simulink model "canal_aquatico_v2"  (R2014a)
settings: Solver=ode45  StartTime=0.0  StopTime=10.0  RelTol=1e-3
libraries: dspsigops x6
settings Model: Creator=andre  LastModifiedBy=andre

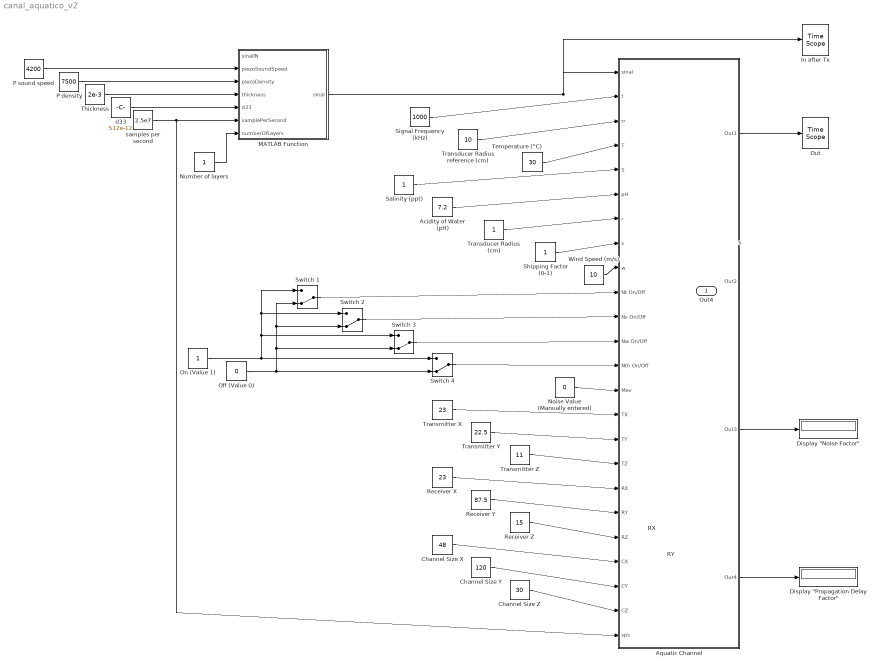
== system canal_aquatico_v2 ==
  s : Inport
  RX : Inport  Port=2
  RY : Inport  Port=3
  Acidity of Water (pH) : Constant  Value=7.2
  Aquatic Channel : Subsystem
  Channel Size X : Constant  Value=48
  Channel Size Y : Constant  Value=120
  Channel Size Z : Constant  Value=30
  "Display \"Propagation Delay Factor\"" : Display
  "Display \"Noise Factor\"" : Display
  In after Tx : TimeScope  DefaultConfigurationName=spbscopes.TimeScopeBlockCfg
  MATLAB Function : MATLAB Function  TreatAsAtomicUnit=on
  Noise Value (Manually entered) : Constant  Value=0
  Number of layers : Constant
  Off (Value 0) : Constant  Value=0
  On (Value 1) : Constant
  Out : TimeScope  DefaultConfigurationName=spbscopes.TimeScopeBlockCfg
  P density : Constant  Value=7500
  P sound speed : Constant  Value=4200
  Receiver X : Constant  Value=23
  Receiver Y : Constant  Value=87.5
  Receiver Z : Constant  Value=15
  Salinity (ppt) : Constant
  Shipping Factor (0-1) : Constant
  Signal Frequency (kHz) : Constant  Value=1000
  Switch {1..4} (4 alike) : ManualSwitch  CurrentSetting=0
  Temperature (°C) : Constant  Value=30
  Thickness : Constant  Value=2e-3
  Transducer Radius (cm) : Constant
  Transducer Radius reference (cm) : Constant  Value=10
  Transmitter X : Constant  Value=23
  Transmitter Y : Constant  Value=22.5
  Transmitter Z : Constant  Value=11
  Wind Speed (m/s) : Constant  Value=10
  d33 : Constant  Value=512e-12
  samples per second : Constant  Value=2.5e7
  Out4 : Outport
  wires:
  MATLAB Function/1(sinal) -> In after Tx/1, Aquatic Channel/1(sinal)
  P sound speed/1 -> MATLAB Function/2(piezoSoundSpeed)
  P density/1 -> MATLAB Function/3(piezoDensity)
  Thickness/1 -> MATLAB Function/4(thickness)
  d33/1 -> MATLAB Function/5(d33)
  samples per second/1 -> Aquatic Channel/24(sps), MATLAB Function/6(samplePerSecond)
  Number of layers/1 -> MATLAB Function/7(numberOfLayers)
  Signal Frequency (kHz)/1 -> Aquatic Channel/2(f)
  Transducer Radius reference (cm)/1 -> Aquatic Channel/3(rr)
  Temperature (°C)/1 -> Aquatic Channel/4(T)
  Salinity (ppt)/1 -> Aquatic Channel/5(S)
  Acidity of Water (pH)/1 -> Aquatic Channel/6(pH)
  Transducer Radius (cm)/1 -> Aquatic Channel/7(r)
  Shipping Factor (0-1)/1 -> Aquatic Channel/8(s)
  Wind Speed (m/s)/1 -> Aquatic Channel/9(w)
  Transmitter X/1 -> Aquatic Channel/15(TX)
  Transmitter Y/1 -> Aquatic Channel/16(TY)
  Transmitter Z/1 -> Aquatic Channel/17(TZ)
  Receiver X/1 -> Aquatic Channel/18(RX)
  Receiver Y/1 -> Aquatic Channel/19(RY)
  Receiver Z/1 -> Aquatic Channel/20(RZ)
  Channel Size X/1 -> Aquatic Channel/21(CX)
  Channel Size Y/1 -> Aquatic Channel/22(CY)
  Channel Size Z/1 -> Aquatic Channel/23(CZ)
  Noise Value (Manually entered)/1 -> Aquatic Channel/14(Mev)
  On (Value 1)/1 -> Switch 1/1, Switch 2/1, Switch 3/1, Switch 4/1
  Off (Value 0)/1 -> Switch 4/2, Switch 1/2, Switch 2/2, Switch 3/2
  Switch 1/1 -> Aquatic Channel/10(Nt On/Off)
  Switch 2/1 -> Aquatic Channel/11(Ns On/Off)
  Switch 3/1 -> Aquatic Channel/12(Nw On/Off)
  Switch 4/1 -> Aquatic Channel/13(Nth On/Off)
  Aquatic Channel/1(Out1) -> Out/1
  Aquatic Channel/3(Out3) -> "Display \"Noise Factor\""/1
  Aquatic Channel/4(Out4) -> "Display \"Propagation Delay Factor\""/1

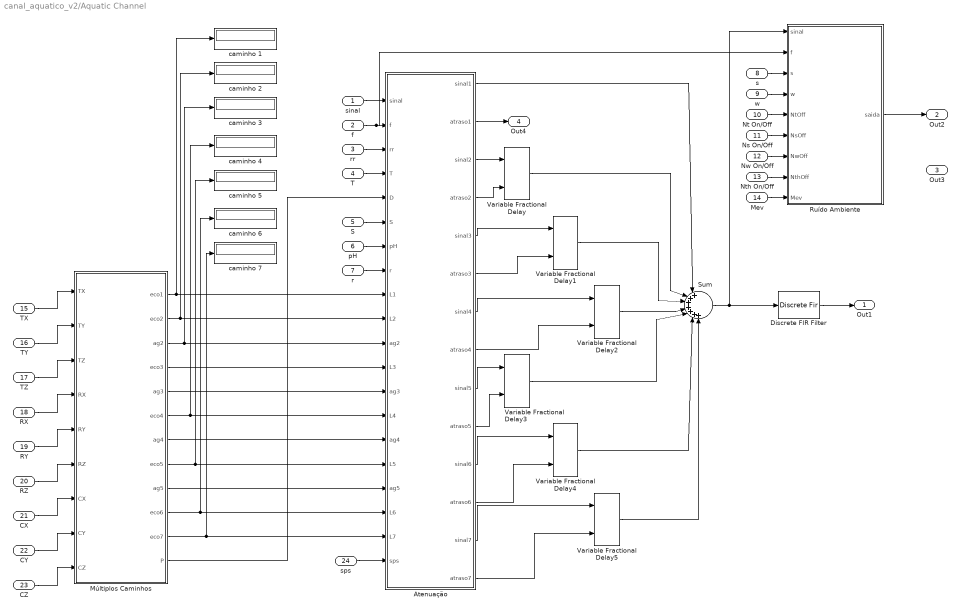
== system canal_aquatico_v2/Aquatic Channel ==
  sinal : Inport
  f : Inport  Port=2
  rr : Inport  Port=3
  T : Inport  Port=4
  S : Inport  Port=5
  pH : Inport  Port=6
  r : Inport  Port=7
  s : Inport  Port=8
  w : Inport  Port=9
  Nt On/Off : Inport  Port=10
  Ns On/Off : Inport  Port=11
  Nw On/Off : Inport  Port=12
  Nth On/Off : Inport  Port=13
  Mev : Inport  Port=14
  TX : Inport  Port=15
  TY : Inport  Port=16
  TZ : Inport  Port=17
  RX : Inport  Port=18
  RY : Inport  Port=19
  RZ : Inport  Port=20
  CX : Inport  Port=21
  CY : Inport  Port=22
  CZ : Inport  Port=23
  sps : Inport  Port=24
  Atenuação : MATLAB Function  TreatAsAtomicUnit=on
  Discrete FIR Filter : DiscreteFir
  Múltiplos Caminhos : MATLAB Function  TreatAsAtomicUnit=on
  Ruído Ambiente : MATLAB Function  TreatAsAtomicUnit=on
  Sum : Sum  Inputs=|+++++++
  Variable Fractional Delay{,1..5} (6 alike) : dspsigops/Variable Fractional Delay  mode=OBSOLETE  modeActive=Linear  dmax=100  InputProcessing=Columns as channels (frame based)  L=4  FarrowL=4  R=10  alpha=1  ic=0  fallbackFIR=Clip to the minimum value necessary for centered kernel  fallbackFarrow=Clip to the minimum value necessary for centered kernel  noDFT=off  roundingMode=Zero  overflowMode=off
  caminho {1..7} (7 alike) : Display
  Out1 : Outport
  Out2 : Outport  Port=2
  Out3 : Outport  Port=3
  Out4 : Outport  Port=4
  wires:
  TX/1 -> Múltiplos Caminhos/1(TX)
  TY/1 -> Múltiplos Caminhos/2(TY)
  TZ/1 -> Múltiplos Caminhos/3(TZ)
  RX/1 -> Múltiplos Caminhos/4(RX)
  RY/1 -> Múltiplos Caminhos/5(RY)
  Múltiplos Caminhos/7(ag4) -> Atenuação/15(ag4)
  f/1 -> Ruído Ambiente/2(f), Atenuação/2(f)
  Múltiplos Caminhos/6(eco4) -> caminho 4/1, Atenuação/14(L4)
  Múltiplos Caminhos/8(eco5) -> caminho 5/1, Atenuação/16(L5)
  Ns On/Off/1 -> Ruído Ambiente/6(NsOff)
  CY/1 -> Múltiplos Caminhos/8(CY)
  Nth On/Off/1 -> Ruído Ambiente/8(NthOff)
  rr/1 -> Atenuação/3(rr)
  Múltiplos Caminhos/10(eco6) -> caminho 6/1, Atenuação/18(L6)
  Múltiplos Caminhos/11(eco7) -> caminho 7/1, Atenuação/19(L7)
  Múltiplos Caminhos/12(P) -> Atenuação/5(D)
  Mev/1 -> Ruído Ambiente/9(Mev)
  S/1 -> Atenuação/6(S)
  Nw On/Off/1 -> Ruído Ambiente/7(NwOff)
  w/1 -> Ruído Ambiente/4(w)
  Nt On/Off/1 -> Ruído Ambiente/5(NtOff)
  Múltiplos Caminhos/9(ag5) -> Atenuação/17(ag5)
  pH/1 -> Atenuação/7(pH)
  Múltiplos Caminhos/4(eco3) -> Atenuação/12(L3)
  Múltiplos Caminhos/5(ag3) -> Atenuação/13(ag3)
  Atenuação/2(atraso1) -> Out4/1
  Múltiplos Caminhos/1(eco1) -> caminho 1/1, Atenuação/9(L1)
  r/1 -> Atenuação/8(r)
  s/1 -> Ruído Ambiente/3(s)
  CZ/1 -> Múltiplos Caminhos/9(CZ)
  RZ/1 -> Múltiplos Caminhos/6(RZ)
  T/1 -> Atenuação/4(T)
  CX/1 -> Múltiplos Caminhos/7(CX)
  sinal/1 -> Atenuação/1(sinal)
  Múltiplos Caminhos/3(ag2) -> caminho 3/1, Atenuação/11(ag2)
  Múltiplos Caminhos/2(eco2) -> caminho 2/1, Atenuação/10(L2)
  Atenuação/9(sinal5) -> Variable Fractional Delay3/1
  Atenuação/7(sinal4) -> Variable Fractional Delay2/1
  Atenuação/13(sinal7) -> Variable Fractional Delay5/1
  Atenuação/8(atraso4) -> Variable Fractional Delay2/2
  Variable Fractional Delay3/1 -> Sum/5
  Atenuação/5(sinal3) -> Variable Fractional Delay1/1
  Atenuação/3(sinal2) -> Variable Fractional Delay/1
  Atenuação/14(atraso7) -> Variable Fractional Delay5/2
  Variable Fractional Delay1/1 -> Sum/3
  Variable Fractional Delay5/1 -> Sum/7
  Atenuação/6(atraso3) -> Variable Fractional Delay1/2
  Atenuação/11(sinal6) -> Variable Fractional Delay4/1
  sps/1 -> Atenuação/20(sps)
  Atenuação/10(atraso5) -> Variable Fractional Delay3/2
  Atenuação/12(atraso6) -> Variable Fractional Delay4/2
  Variable Fractional Delay/1 -> Sum/2
  Atenuação/1(sinal1) -> Sum/1
  Atenuação/4(atraso2) -> Variable Fractional Delay/2
  Variable Fractional Delay2/1 -> Sum/4
  Variable Fractional Delay4/1 -> Sum/6
  Sum/1 -> Discrete FIR Filter/1, Ruído Ambiente/1(sinal)
  Discrete FIR Filter/1 -> Out1/1
  Ruído Ambiente/1(saida) -> Out2/1

== matlab function canal_aquatico_v2/Aquatic Channel/Atenuação ==
  data: sinal input; f input; rr input; T input; D input; S input; pH input; r input; sinal1 output; L1 input; L2 input; ag2 input; L3 input; ag3 input; L4 input; ag4 input; L5 input; ag5 input; L6 input; L7 input; sps input; atraso1 output; sinal2 output; atraso2 output; sinal3 output; atraso3 output; sinal4 output; atraso4 output; sinal5 output; atraso5 output; sinal6 output; atraso6 output; sinal7 output; atraso7 output
%Bloc attenuation

%Function Definition
function [sinal1,atraso1,sinal2,atraso2,sinal3,atraso3,sinal4,atraso4,sinal5,atraso5,sinal6,atraso6,sinal7,atraso7]  = bloco_atenuacao(sinal,f,rr,T,D,S,pH,r,L1,L2,ag2,L3,ag3,L4,ag4,L5,ag5,L6,L7,sps)

%Parameter Values (Boric Acid and Magnesium Sulphate)
f1 = 0.78 * sqrt(S/35) * (exp(T/26));
f2 = 42 * (exp(T/17));

%Speed of sound (m/s)
cmetro = 1448.96 + 4.591*T - 5.304*(10^(-2))*(T^(2)) +...
    + 2.374*(10^(-4))*(T^(3))...
    + 1.340*(S-35) + 1.630*(10^(-2))*D + 1.675*(10^(-7))*(D^(2)) +...
    - 1.025*(10^(-2))*T*(S-35) - 7.139*(10^(-13))*T*(D^(3));

%Conversion from m/s to cm/s
c=cmetro*100;

%Calculation of wavelength
lambda = c/(f*1000);

%Calculation of the transducer diameter
angulo = 0;
d = 2*r;
de = (pi*rr^2);

%Absorption Coefficient
a = ((0.106 * (f1 * f^2) * exp((pH - 8)/0.56)) / (f1^2 + f^2)) +...
    ((0.52 * (1 + (T/43)) * (S/45) * (f2 * f^2) *...
    exp(-(D/6))) / (f2^2 + f^2)) + (0.00049 * (f^2) * (exp(-(T/27 + D/17))));

%Attenuation
ab1 = a*(L1/1e5);

ab2 = a*(L2/1e5);

ab3 = a*(L3/1e5);

ab4 = a*(L4/1e5);

ab5 = a*(L5/1e5);

ab6 = a*(L6/1e5);

ab7 = a*(L7/1e5);

if  r < lambda;
    angulo = pi/2;
end
if  r > lambda;
    angulo = asin(lambda/d);
end

sp1 = 10*log10(((2*angulo*(L1)^2) + de)/de);
sp2 = 10*log10(((2*angulo*(L2)^2) + de)/de);
sp3 = 10*log10(((2*angulo*(L3)^2) + de)/de);
sp4 = 10*log10(((2*angulo*(L4)^2) + de)/de);
sp5 = 10*log10(((2*angulo*(L5)^2) + de)/de);
sp6 = 10*log10(((2*angulo*(L6)^2) + de)/de);
sp7 = 10*log10(((2*angulo*(L7)^2) + de)/de);

sinal1 = 0;
sinal2 = 0;
sinal3 = 0;
sinal4 = 0;
sinal5 = 0;
sinal6 = 0;
sinal7 = 0;

atraso1=0;
atraso2=0;
atraso3=0;
atraso4=0;
atraso5=0;
atraso6=0;
atraso7=0;

sinal1= 10^((-1*(ab1 + sp1))/10);
atraso1= ((L1/c)*sps);

%if(ag2<=angulo)
sinal2= 10^((-1*(ab2 + sp2))/10);
atraso2= ((L2/c)*sps)-at1;
%end
%if(ag3<=angulo)
sinal3 = 10^((-1*(ab3 + sp3))/10);
atraso3= ((L3/c)*sps)-at1;
%end
%if(ag4<=angulo)
sinal4 = 10^((-1*(ab4 + sp4))/10);
atraso4= ((L4/c)*sps)-at1;
%end
%if(ag5<=angulo)
sinal5 = 10^((-1*(ab5 + sp5))/10);
atraso5= ((L5/c)*sps)-at1;
%end
if (L6>0)
    sinal6 = 10^((-1*(ab6 + sp6))/10);
    atraso6= ((L6/c)*sps)-at1;
end
if (L7>0)
    sinal7 = 10^((-1*(ab7 + sp7))/10);
    atraso7= ((L7/c)*sps)-at1;
end

atraso1=atraso1/sps;
%agT=angulo;

== matlab function canal_aquatico_v2/Aquatic Channel/Múltiplos Caminhos ==
  data: TX input; eco1 output; TY input; TZ input; RX input; RY input; RZ input; CX input; CY input; CZ input; eco2 output; ag2 output; eco3 output; ag3 output; eco4 output; ag4 output; eco5 output; ag5 output; eco6 output; eco7 output; P output
function [eco1,eco2,ag2,eco3,ag3,eco4,ag4,eco5,ag5,eco6,eco7,P] = bloco_multiplos(TX,TY,TZ,RX,RY,RZ,CX,CY,CZ)



eco1 = sqrt((RX-TX)^2 + (RY-TY)^2 + (RZ-TZ)^2);

eco2 = sqrt( ((2*CX-RX)-TX)^2 + (RY-TY)^2 + (RZ-TZ)^2 );

ag2 = asin(abs((2*CX-RX)-TX)/eco2);

eco3 = sqrt( (-RX-TX)^2 + (RY-TY)^2 + (RZ-TZ)^2 );

ag3 = asin((RX+TX)/eco3);

eco4 = sqrt( (RX-TX)^2 + (RY-TY)^2 + ((2*CZ-RZ)-TZ)^2 );

ag4 = asin(abs((2*CZ-RZ)-TZ)/eco4);

eco5 = sqrt( (RX-TX)^2 + (RY-TY)^2 + (-RZ-TZ)^2 );

ag5 = asin((RZ+TZ)/eco5);

if((RZ==TZ) && (RX==TX))
    eco6 = (RY+TY);
    eco7 = sqrt(((2*CY-RY)-TY)^2);
else
    eco6 = 0;
    eco7 = 0;
end

P=(RZ+TZ)/2;

== matlab function canal_aquatico_v2/Aquatic Channel/Ruído Ambiente ==
  data: sinal input; f input; saida output; s input; w input; NtOff input; NsOff input; NwOff input; NthOff input; Mev input
function saida = bloco_ruido_ambiente (sinal,f,s,w,NtOff,NsOff,NwOff,NthOff,Mev)
% f - signal frequency (kHz); 
% s - shipping factor (between 0 - 1);
% w - wind speed (m/s); 
% NtOff, NsOff, NwOff, NthOff - Disable the corresponding equation;
% Mev - Manually entered value.

%Equation of Turbulence Noise
Nt = (10^((17-30*log10(f))/10))*NtOff;

%Equation of Shipping Noise
Ns = (10^((40+(20*(s-0.5))+(26*log10(f))-(60*log10(f+0.03)))/10))*NsOff;

%Equation of Wave Noise
Nw = (10^((50+(7.5*(w^(1/2)))+(20*log10(f))-(40*log10(f+0.4)))/10))*NwOff;

%Equation of Thermal Noise
Nth = (10^((-15+20*log10(f))/10))*NthOff;

%Total Noise
saida = Nt + Ns + Nw + Nth + Mev;

== matlab function canal_aquatico_v2/MATLAB Function ==
  data: sinalIN input; sinal output; piezoSoundSpeed input; piezoDensity input; thickness input; d33 input; samplePerSecond input; numberOfLayers input
function sinal = projetor(sinalIN, piezoSoundSpeed, piezoDensity, thickness, d33, samplePerSecond, numberOfLayers)

%A simulação realizada nesse bloco é feita no Software COMSOL.
% fr é o range da frequencia de ressonancia 
% f é a frequencia selecionada dentro do range
%fr = [16090 ,19800];

f1 = 16090;
%f2 = 19800;
% todo -  explicar frequencia de amostragem
Ts = 1/(2*1000000);
t=0:Ts:1000*Ts;
sinal = 12*(sin(2*pi*f1*t));
%plot(t,sinal);
